simulink library "sy202_elevator_library"  (R2015a)
settings: Solver=ode45  StartTime=0.0  StopTime=10.0  RelTol=1e-3
libraries: simulink x1
settings Model: Creator=DeVries  LastModifiedBy=devries

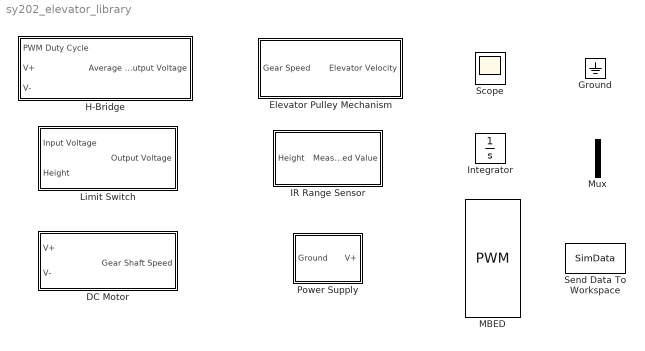
== system sy202_elevator_library ==
  DC Motor : Subsystem  mask(DC Motor){ktb=0.0477, Je=1.0081e-05, Td=0.0029}
      mask prompts: ktb "Transducer Constant"; Je "Moment of Inertia"; Td "Static Friction"
      mask help:
      | This block represents the dynamics of a direct current motor. The motor has
      | positive and negative voltage input leads and generates the angular
      | velocity of the motor:
      |
      | Inputs:
      |         V+ = Positive reference voltage
      |         V- = Negative reference voltage
      |
      | Output:
      |         Gear Shaft Speed = the rate of rotation of the motor shaft in
      |         rad/s
  Elevator Pulley Mechanism : Subsystem  mask{r_p=0.2015}
      mask prompts: r_p "Pulley Radius"
  Ground : Ground
  H-Bridge : Subsystem  mask(H-Bridge){}
      mask help:
      | The H-bridge block enables control of a DC motor. The H-bridge modifies the voltage level to the DC motor operating voltage switches the current flow to allow directional control.
      |
      | Inputs:
      |     PWM duty cycle: The duty cycle of the PWM motor control signal (from mbed).
      |     V+:             Positive reference voltage
      |     V-:             Negative reference voltage
      |
      | Outputs:
      |     Average Output Voltage: Scaled voltage signal
  IR Range Sensor : Subsystem  mask(Infrared Sensor){noisPow=0.0001}
      mask prompts: noisPow "Noise Magnitude"
      mask help: The block models an infrared range sensor.
  Integrator : Integrator
  Limit Switch : Subsystem  mask(Elevator Limit Switch(es)){maxHeight=27.125, minHeight=5.75}
      mask prompts: maxHeight "Maximum Height"; minHeight "Minimum Height"
      mask help:
      | This block models the funcitonality of the limit switches on the ES202 elevator setup.  If the height of the elevator car is greater than XX inches or less than YY inches the limit switches are open. Otherwise, the switches are closed.
      |
      | Inputs:
      |         Input Voltage = Voltage into the switch
      |         Height = Height of the elevator car
      |
      | Outputs:
      |         Output Voltage = Voltage on the output side of the switch
      |
      | The parameters set the maximum and minimum heights that open the switches.
  MBED : Constant  Value=PWM  mask{PWM=0.5}
      mask prompts: PWM "PWM Duty Cycle"
      mask Display: image(imread('mbed.jpeg'))
  Mux : Mux  Inputs=2
  Power Supply : Subsystem  mask(Power Supply){Vsupply=12}
      mask prompts: Vsupply "Voltage Change"
      mask help:
      | This block models the voltage produced by the power supply. The power supply increases the output voltage above the local ground by an amount specified in the parameter block.
      |
      | Inputs:
      |         Ground = local ground (0 Volts typically)
      |
      | Output:
      |         V+ = output voltage above local ground
      |
      | Parameter:
      |         Voltage Change = Change in voltage generated by the power supply
  Scope : Scope
  Send Data To Workspace : ToWorkspace  VariableName=SimData  SaveFormat=Structure With Time  SampleTime=-1

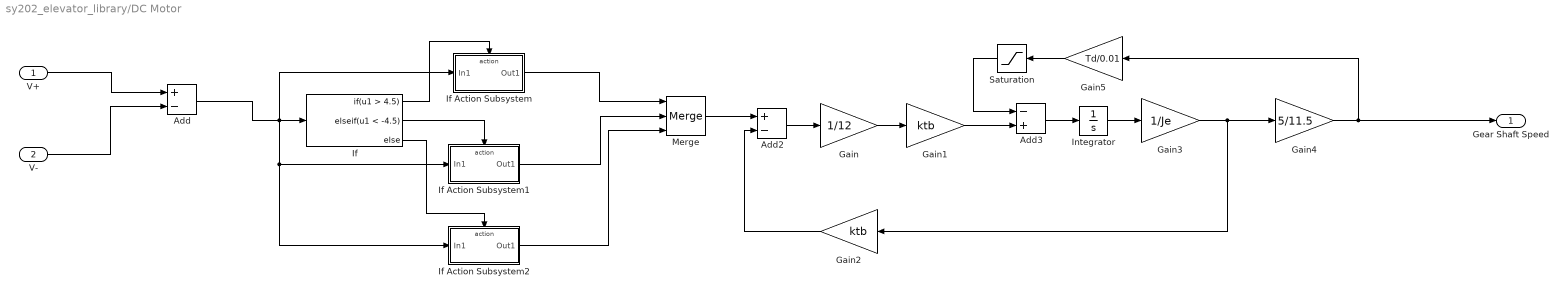
== system sy202_elevator_library/DC Motor ==
  V+ : Inport
  V- : Inport  Port=2
  Add : Sum  Inputs=+-
  Add2 : Sum  Inputs=+-
  Add3 : Sum  Inputs=-+
  Gain : Gain  Gain=1/12
  Gain1 : Gain  Gain=ktb
  Gain2 : Gain  Gain=ktb
  Gain3 : Gain  Gain=1/Je
  Gain4 : Gain  Gain=5/11.5
  Gain5 : Gain  Gain=Td/0.01
  If : If  IfExpression=u1 > 4.5  ElseIfExpressions=u1 < -4.5
  If Action Subsystem : Subsystem  TreatAsAtomicUnit=on
  If Action Subsystem1 : Subsystem  TreatAsAtomicUnit=on
  If Action Subsystem2 : Subsystem  TreatAsAtomicUnit=on
  Integrator : Integrator
  Merge : Merge  Inputs=3
  Saturation : Saturate  UpperLimit=Td  LowerLimit=-Td
  Gear Shaft Speed : Outport
  wires:
  Add/1 -> If Action Subsystem/1(In1), If Action Subsystem1/1(In1), If Action Subsystem2/1(In1), If/1
  Merge/1 -> Add2/1
  If/3 -> If Action Subsystem2/Action
  If/1 -> If Action Subsystem/Action
  If Action Subsystem2/1(Out1) -> Merge/3
  If Action Subsystem1/1(Out1) -> Merge/2
  If Action Subsystem/1(Out1) -> Merge/1
  If/2 -> If Action Subsystem1/Action
  V+/1 -> Add/1
  V-/1 -> Add/2
  Add2/1 -> Gain/1
  Gain/1 -> Gain1/1
  Integrator/1 -> Gain3/1
  Gain3/1 -> Gain2/1, Gain4/1
  Gain1/1 -> Add3/2
  Saturation/1 -> Add3/1
  Gain5/1 -> Saturation/1
  Gain2/1 -> Add2/2
  Add3/1 -> Integrator/1
  Gain4/1 -> Gear Shaft Speed/1, Gain5/1

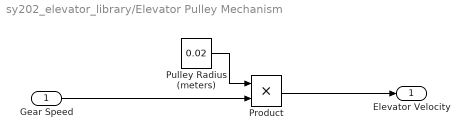
== system sy202_elevator_library/Elevator Pulley Mechanism ==
  Gear Speed : Inport
  Product : Product
  Pulley Radius (meters) : Constant  Value=0.02
  Elevator Velocity : Outport
  wires:
  Gear Speed/1 -> Product/2
  Pulley Radius (meters)/1 -> Product/1
  Product/1 -> Elevator Velocity/1

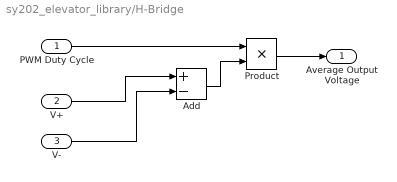
== system sy202_elevator_library/H-Bridge ==
  PWM Duty Cycle : Inport
  V+ : Inport  Port=2
  V- : Inport  Port=3
  Add : Sum  Inputs=+-
  Product : Product
  Average Output Voltage : Outport
  wires:
  Product/1 -> Average Output Voltage/1
  PWM Duty Cycle/1 -> Product/1
  Add/1 -> Product/2
  V+/1 -> Add/1
  V-/1 -> Add/2

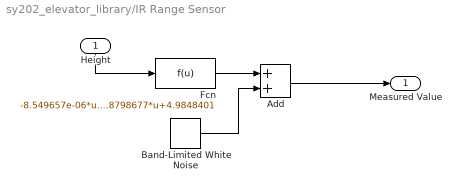
== system sy202_elevator_library/IR Range Sensor ==
  Height : Inport
  Add : Sum
  Band-Limited White Noise : simulink/Sources/Band-Limited White Noise  Cov=[noisPow]  Ts=0.1  seed=[23341]
  Fcn : Fcn  Expr=-8.549657e-06*u^5+.000662389*u^4-0.0196244*u^3+0.278528*u^2-1.8798677*u+4.9848401
  Measured Value : Outport
  wires:
  Add/1 -> Measured Value/1
  Band-Limited White Noise/1 -> Add/2
  Fcn/1 -> Add/1
  Height/1 -> Fcn/1

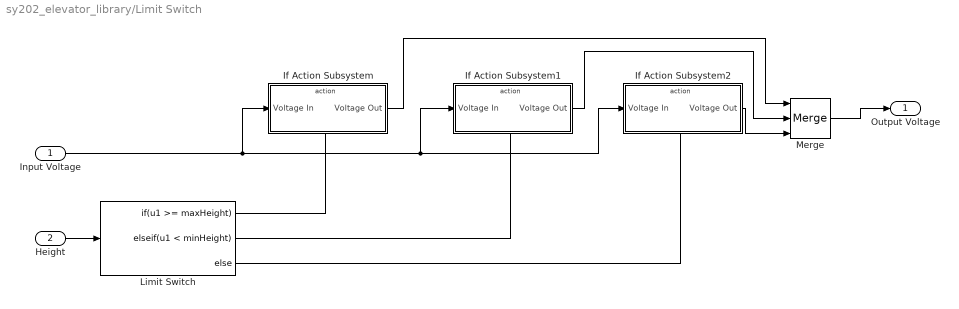
== system sy202_elevator_library/Limit Switch ==
  Input Voltage : Inport
  Height : Inport  Port=2
  If Action Subsystem : Subsystem  TreatAsAtomicUnit=on
  If Action Subsystem1 : Subsystem  TreatAsAtomicUnit=on
  If Action Subsystem2 : Subsystem  TreatAsAtomicUnit=on
  Limit Switch : If  IfExpression=u1 >= maxHeight  ElseIfExpressions=u1 < minHeight
  Merge : Merge  Inputs=3
  Output Voltage : Outport
  wires:
  Height/1 -> Limit Switch/1
  Input Voltage/1 -> If Action Subsystem2/1(Voltage In), If Action Subsystem1/1(Voltage In), If Action Subsystem/1(Voltage In)
  Limit Switch/3 -> If Action Subsystem2/Action
  Limit Switch/2 -> If Action Subsystem1/Action
  Limit Switch/1 -> If Action Subsystem/Action
  If Action Subsystem/1(Voltage Out) -> Merge/1
  If Action Subsystem1/1(Voltage Out) -> Merge/2
  If Action Subsystem2/1(Voltage Out) -> Merge/3
  Merge/1 -> Output Voltage/1

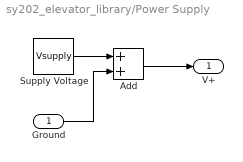
== system sy202_elevator_library/Power Supply ==
  Ground : Inport
  Add : Sum
  Supply Voltage : Constant  Value=Vsupply
  V+ : Outport
  wires:
  Supply Voltage/1 -> Add/1
  Add/1 -> V+/1
  Ground/1 -> Add/2

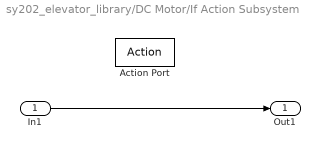
== system sy202_elevator_library/DC Motor/If Action Subsystem ==
  In1 : Inport
  Action Port : ActionPort
  Out1 : Outport
  wires:
  In1/1 -> Out1/1

== system sy202_elevator_library/DC Motor/If Action Subsystem1 ==
  In1 : Inport
  Action Port : ActionPort
  Out1 : Outport
  wires:
  In1/1 -> Out1/1

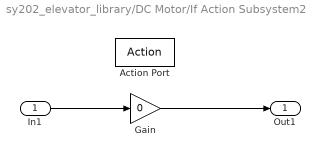
== system sy202_elevator_library/DC Motor/If Action Subsystem2 ==
  In1 : Inport
  Action Port : ActionPort
  Gain : Gain  Gain=0
  Out1 : Outport
  wires:
  In1/1 -> Gain/1
  Gain/1 -> Out1/1

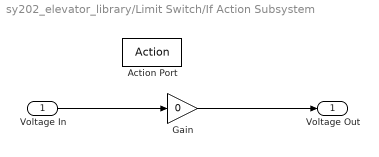
== system sy202_elevator_library/Limit Switch/If Action Subsystem ==
  Voltage In : Inport
  Action Port : ActionPort
  Gain : Gain  Gain=0
  Voltage Out : Outport
  wires:
  Voltage In/1 -> Gain/1
  Gain/1 -> Voltage Out/1

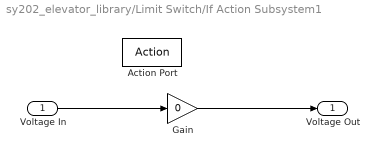
== system sy202_elevator_library/Limit Switch/If Action Subsystem1 ==
  Voltage In : Inport
  Action Port : ActionPort
  Gain : Gain  Gain=0
  Voltage Out : Outport
  wires:
  Voltage In/1 -> Gain/1
  Gain/1 -> Voltage Out/1

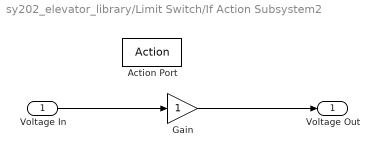
== system sy202_elevator_library/Limit Switch/If Action Subsystem2 ==
  Voltage In : Inport
  Action Port : ActionPort
  Gain : Gain
  Voltage Out : Outport
  wires:
  Voltage In/1 -> Gain/1
  Gain/1 -> Voltage Out/1
